simulink model "Assignment3"  (R2014a)
settings: Solver=FixedStepDiscrete  StartTime=0.0  StopTime=300000  FixedStep=1  RelTol=1e-3
libraries: hdlsllib x3, simulink x2
settings Model: Creator=vu.du  LastModifiedBy=vu.du

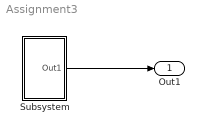
== system Assignment3 ==
  Subsystem : Subsystem  TreatAsAtomicUnit=on
  Out1 : Outport
  wires:
  Subsystem/1(Out1) -> Out1/1

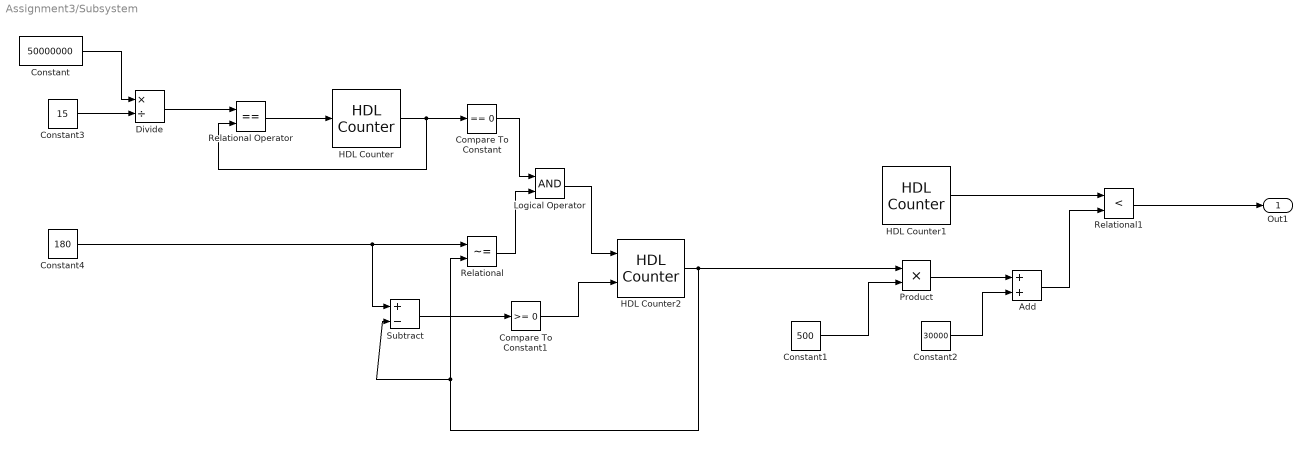
== system Assignment3/Subsystem ==
  Add : Sum
  Compare To Constant : simulink/Logic and Bit Operations/Compare To Constant  relop===  const=0  OutDataTypeStr=boolean
  Compare To Constant1 : simulink/Logic and Bit Operations/Compare To Constant  relop=>=  const=0  OutDataTypeStr=boolean
  Constant : Constant  Value=50000000  OutDataTypeStr=int32
  Constant1 : Constant  Value=500  OutDataTypeStr=int32
  Constant2 : Constant  Value=30000  OutDataTypeStr=int32
  Constant3 : Constant  Value=15  OutDataTypeStr=int8  SampleTime=1
  Constant4 : Constant  Value=180  OutDataTypeStr=int32  SampleTime=1
  Divide : Product  Inputs=*/  OutDataTypeStr=int32  SaturateOnIntegerOverflow=on  RndMeth=Zero
  HDL Counter : hdlsllib/HDL Operations/HDL Counter  CountType=Free running  CountInit=0  CountStep=1  CountMax=100  CountFromType=Initial value  CountFrom=0  CountResetPort=on  CountLoadPort=off  CountEnbPort=off  CountDirPort=off  CountDataType=Unsigned  CountWordLen=32  CountFracLen=0  CountSampTime=1
  HDL Counter1 : hdlsllib/HDL Operations/HDL Counter  CountType=Count limited  CountInit=0  CountStep=1  CountMax=1000000  CountFromType=Initial value  CountFrom=0  CountResetPort=off  CountLoadPort=off  CountEnbPort=off  CountDirPort=off  CountDataType=Unsigned  CountWordLen=32  CountFracLen=0  CountSampTime=1
  HDL Counter2 : hdlsllib/HDL Operations/HDL Counter  CountType=Count limited  CountInit=90  CountStep=1  CountMax=180  CountFromType=Specify  CountFrom=0  CountResetPort=off  CountLoadPort=off  CountEnbPort=on  CountDirPort=on  CountDataType=Unsigned  CountWordLen=32  CountFracLen=0  CountSampTime=1
  Logical Operator : Logic  AllPortsSameDT=off  OutDataTypeStr=boolean
  Product : Product
  Relational : RelationalOperator  Operator=~=  OutDataTypeStr=boolean
  Relational Operator : RelationalOperator  Operator===  OutDataTypeStr=boolean
  Relational1 : RelationalOperator  Operator=<  OutDataTypeStr=boolean
  Subtract : Sum  Inputs=+-
  Out1 : Outport
  wires:
  Relational/1 -> Logical Operator/2
  Divide/1 -> Relational Operator/1
  HDL Counter/1 -> Relational Operator/2, Compare To Constant/1
  Constant/1 -> Divide/1
  Constant3/1 -> Divide/2
  Relational Operator/1 -> HDL Counter/1
  Subtract/1 -> Compare To Constant1/1
  Product/1 -> Add/1
  Compare To Constant1/1 -> HDL Counter2/2
  Constant2/1 -> Add/2
  Add/1 -> Relational1/2
  HDL Counter2/1 -> Product/1, Subtract/2, Relational/2
  Relational1/1 -> Out1/1
  Logical Operator/1 -> HDL Counter2/1
  Compare To Constant/1 -> Logical Operator/1
  HDL Counter1/1 -> Relational1/1
  Constant4/1 -> Subtract/1, Relational/1
  Constant1/1 -> Product/2
